simulink subsystem "CombinedConverterSub"  (R2025a)
settings: Solver=VariableStepAuto  StartTime=0.0  StopTime=10.0  RelTol=1e-3
settings Model: Creator=james  LastModifiedBy=james

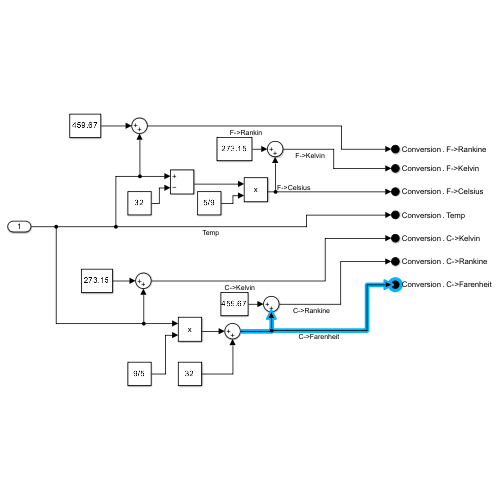
[thumbnail: Simulink's stored preview of the top-level diagram]
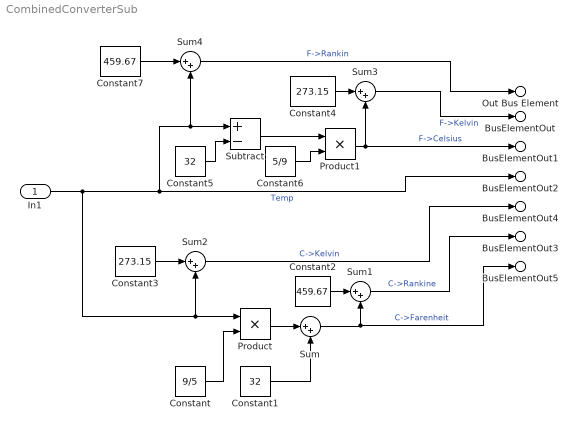
== system CombinedConverterSub ==
  In1 : Inport
  Constant : Constant  Value=9/5
  Constant1 : Constant  Value=32
  Constant2 : Constant  Value=459.67
  Constant3 : Constant  Value=273.15
  Constant4 : Constant  Value=273.15
  Constant5 : Constant  Value=32
  Constant6 : Constant  Value=5/9
  Constant7 : Constant  Value=459.67
  Product : Product
  Product1 : Product
  Subtract : Sum  Inputs=+-
  Sum{,1..4} (5 alike) : Sum  Inputs=|++
  Out Bus Element : Outport  PortName=Conversion  Element=F->Rankine
  BusElementOut : Outport  PortName=Conversion  Element=F->Kelvin
  BusElementOut1 : Outport  PortName=Conversion  Element=F->Celsius
  BusElementOut2 : Outport  PortName=Conversion  Element=Temp
  BusElementOut3 : Outport  PortName=Conversion  Element=C->Rankine
  BusElementOut4 : Outport  PortName=Conversion  Element=C->Kelvin
  BusElementOut5 : Outport  PortName=Conversion  Element=C->Farenheit
  wires:
  Constant/1 -> Product/2
  Product/1 -> Sum/1
  Constant2/1 -> Sum1/1
  Sum1/1 -> BusElementOut3/1  "C->Rankine"
  Sum2/1 -> BusElementOut4/1  "C->Kelvin"
  Sum/1 -> BusElementOut5/1, Sum1/2  "C->Farenheit"
  Constant1/1 -> Sum/2
  Constant3/1 -> Sum2/1
  In1/1 -> Sum2/2, Product/1, BusElementOut2/1, Sum4/2, Subtract/1  "Temp"
  Sum4/1 -> Out Bus Element/1  "F->Rankin"
  Sum3/1 -> BusElementOut/1  "F->Kelvin"
  Constant7/1 -> Sum4/1
  Subtract/1 -> Product1/1
  Constant4/1 -> Sum3/1
  Product1/1 -> BusElementOut1/1, Sum3/2  "F->Celsius"
  Constant5/1 -> Subtract/2
  Constant6/1 -> Product1/2
